simulink model "fft_filter"  (R2024a)
settings: Solver=VariableStepAuto  StartTime=0.0  StopTime=10.0  RelTol=1e-3
values from neighbouring files (symbols this model uses):
  b = fir1(numtaps-1, fc/(fs/2), 'low', hamming(numtaps))    [param_for_fir_fft.m]
libraries: dspxfrm3 x1, dspspect3 x1
settings Model: Creator=MaxV  LastModifiedBy=MaxV

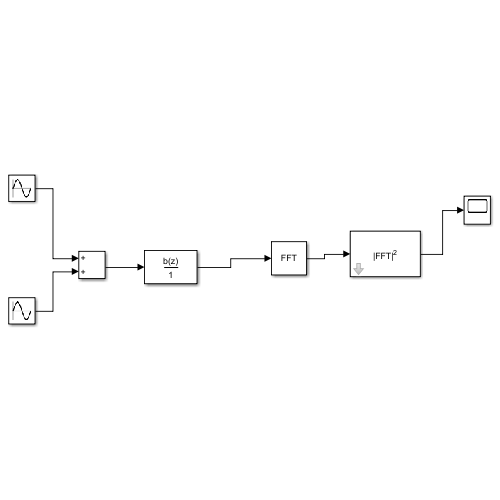
[thumbnail: Simulink's stored preview of the top-level diagram]
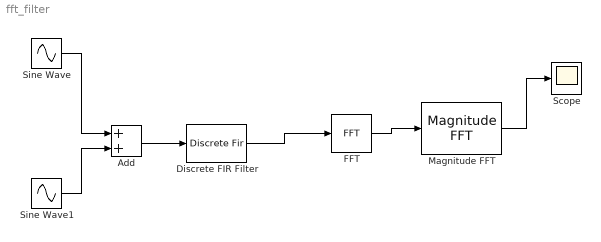
== system fft_filter ==
  Add : Sum
  Discrete FIR Filter : DiscreteFir  Coefficients=b
  FFT : dspxfrm3/FFT  FFTImplementation=Auto  CompMethod=Table lookup  TableOpt=NEW  TableOptActive=Speed  BitRevOrder=off  Normalize=off  InheritFFTLength=on  FFTLength=64  WrapInput=on  roundingMode=Ceiling  overflowMode=off  firstCoeffDataTypeStr=Inherit: Same word length as input  firstCoeffLastDataTypeStr=Inherit: Same word length as input  outputMin=[]  outputMax=[]
  Magnitude FFT : dspspect3/Magnitude FFT  mag_or_magsq=Magnitude squared  FFTImplementation=Auto  fftLenInherit=off  fftsize=256  WrapInput=on
  Scope : Scope
  Sine Wave : Sin  Frequency=2*pi*50  SampleTime=0
  Sine Wave1 : Sin  Amplitude=0.5  Frequency=2*pi*120  SampleTime=0
  wires:
  Sine Wave/1 -> Add/1
  Sine Wave1/1 -> Add/2
  Add/1 -> Discrete FIR Filter/1
  Discrete FIR Filter/1 -> FFT/1
  FFT/1 -> Magnitude FFT/1
  Magnitude FFT/1 -> Scope/1
